simulink model "GT_L1"  (R2024a)
settings: Solver=ode4  StartTime=0.0  StopTime=500  FixedStep=1/1600  RelTol=1e-3
undefined symbols (not defined in the file): G_L1, RLL_Freq
libraries: aerolibactuator x2, AP_RollController x1, AP_YawController x1
settings Model: Creator=igmso  LastModifiedBy=igmso
settings DataIOCC: ExternalInput=[t,u]  InitialState=getstatestruct(op_trim3)  SaveFormat=StructureWithTime

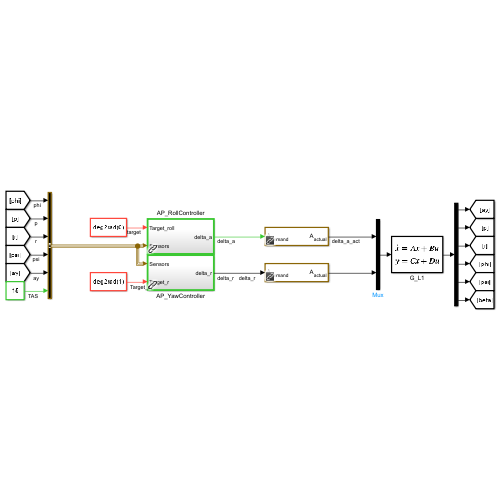
[thumbnail: Simulink's stored preview of the top-level diagram]
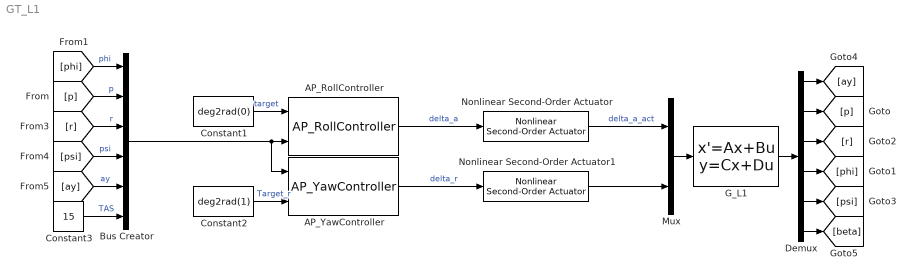
== system GT_L1 ==
  AP_RollController : AP_RollController/AP_RollController  SystemSampleTime=1/RLL_Freq  VariantActivationTime=update diagram  AllowFlexibleInterface=on  Latency=0  AutoFrameSizeCalculation=off
  AP_YawController : AP_YawController/AP_YawController  SystemSampleTime=1/RLL_Freq  VariantActivationTime=update diagram  AllowFlexibleInterface=on  Latency=0  AutoFrameSizeCalculation=off
  Bus Creator : BusCreator  Inputs=6
  Constant1 : Constant  Value=deg2rad(0)  SampleTime=-1
  Constant2 : Constant  Value=deg2rad(1)  SampleTime=-1
  Constant3 : Constant  Value=15  SampleTime=-1
  Demux : Demux  Outputs=6
  G_L1 : StateSpace  A=G_L1.A  B=G_L1.B  C=G_L1.C  D=G_L1.D  InitialCondition=0  ContinuousStateAttributes=G_L1.StateName
  Mux : Mux  Inputs=2
  Nonlinear Second-Order Actuator : aerolibactuator/Nonlinear Second-Order Actuator  wn_fin=2  z_fin=0.7  fin_max=15  fin_min=-15  fin_maxrate=400  fin_act_0=0  fin_act_vel=0
  Nonlinear Second-Order Actuator1 : aerolibactuator/Nonlinear Second-Order Actuator  wn_fin=2  z_fin=0.7  fin_max=15  fin_min=-15  fin_maxrate=400  fin_act_0=0  fin_act_vel=0
  wires:
  Mux/1 -> G_L1/1
  Nonlinear Second-Order Actuator1/1 -> Mux/2
  G_L1/1 -> Demux/1
  Bus Creator/1 -> AP_YawController/1, AP_RollController/2
  [phi] -> Bus Creator/1  "phi"
  [p] -> Bus Creator/2  "p"
  Demux/1 -> [ay]
  Demux/3 -> [r]
  Demux/6 -> [beta]
  Demux/2 -> [p]
  Demux/4 -> [phi]
  Constant1/1 -> AP_RollController/1  "target"
  AP_RollController/1 -> Nonlinear Second-Order Actuator/1  "delta_a"
  Nonlinear Second-Order Actuator/1 -> Mux/1  "delta_a_act"
  Demux/5 -> [psi]
  [r] -> Bus Creator/3  "r"
  [psi] -> Bus Creator/4  "psi"
  [ay] -> Bus Creator/5  "ay"
  Constant3/1 -> Bus Creator/6  "TAS"
  AP_YawController/1 -> Nonlinear Second-Order Actuator1/1  "delta_r"
  Constant2/1 -> AP_YawController/2  "Target_r"
